simulink model "prob4"  (R2020b)
settings: Solver=VariableStepAuto  StartTime=0.0  StopTime=10.0  RelTol=1e-3
undefined symbols (not defined in the file or in its folder): b, J, Ke, Kt, L, R
settings Model: DataDictionary=data4.sldd  Creator=deves  LastModifiedBy=deves

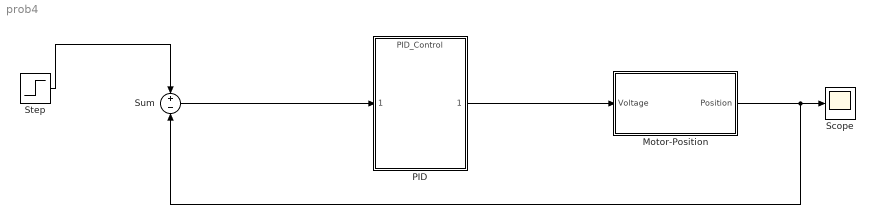
== system prob4 ==
  Motor-Position : Subsystem
  PID : ModelReference  ModelNameDialog=PID_Control  SimulationMode=Normal  ModelReferenceVersion=1.1
  Scope : Scope
  Step : Step  SampleTime=0
  Sum : Sum  Inputs=+-
  wires:
  Motor-Position/1(Position) -> Sum/2, Scope/1
  PID/1 -> Motor-Position/1(Voltage)
  Step/1 -> Sum/1
  Sum/1 -> PID/1

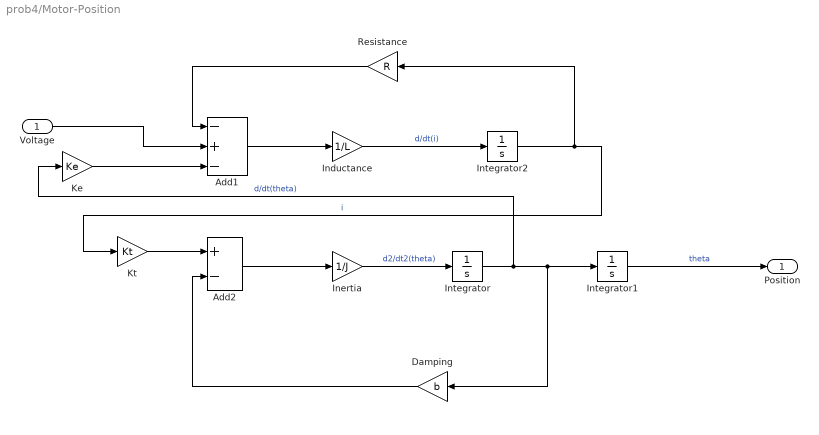
== system prob4/Motor-Position ==
  Voltage : Inport  OutDataTypeStr=double  PortDimensions=1  SampleTime=0
  Add1 : Sum  Inputs=-+-
  Add2 : Sum  Inputs=+-
  Damping : Gain  Gain=b
  Inductance : Gain  Gain=1/L
  Inertia : Gain  Gain=1/J
  Integrator : Integrator
  Integrator1 : Integrator
  Integrator2 : Integrator
  Ke : Gain  Gain=Ke
  Kt : Gain  Gain=Kt
  Resistance : Gain  Gain=R
  Position : Outport  OutDataTypeStr=double  PortDimensions=1  SampleTime=0
  wires:
  Integrator/1 -> Integrator1/1, Damping/1, Ke/1  "d/dt(theta)"
  Kt/1 -> Add2/1
  Add1/1 -> Inductance/1
  Integrator1/1 -> Position/1  "theta"
  Add2/1 -> Inertia/1
  Damping/1 -> Add2/2
  Ke/1 -> Add1/3
  Inertia/1 -> Integrator/1  "d2/dt2(theta)"
  Voltage/1 -> Add1/2
  Inductance/1 -> Integrator2/1  "d/dt(i)"
  Integrator2/1 -> Kt/1, Resistance/1  "i"
  Resistance/1 -> Add1/1
